simulink model "Uni_Canberra_Inverted_Pendulum"  (R2025b)
settings: Solver=FixedStepDiscrete  StartTime=0  StopTime=50  FixedStep=0.1  RelTol=1e-3
settings Model: Creator=s445788  LastModifiedBy=s445788

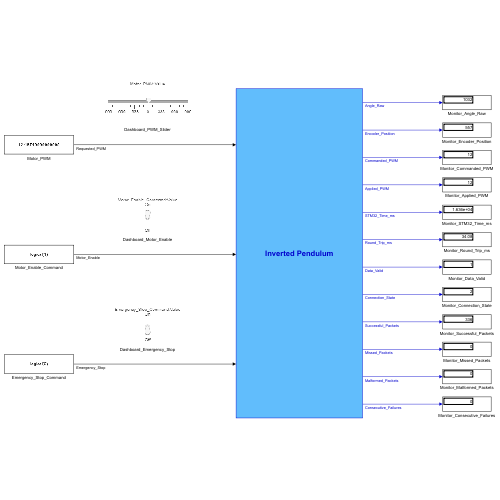
[thumbnail: Simulink's stored preview of the top-level diagram]
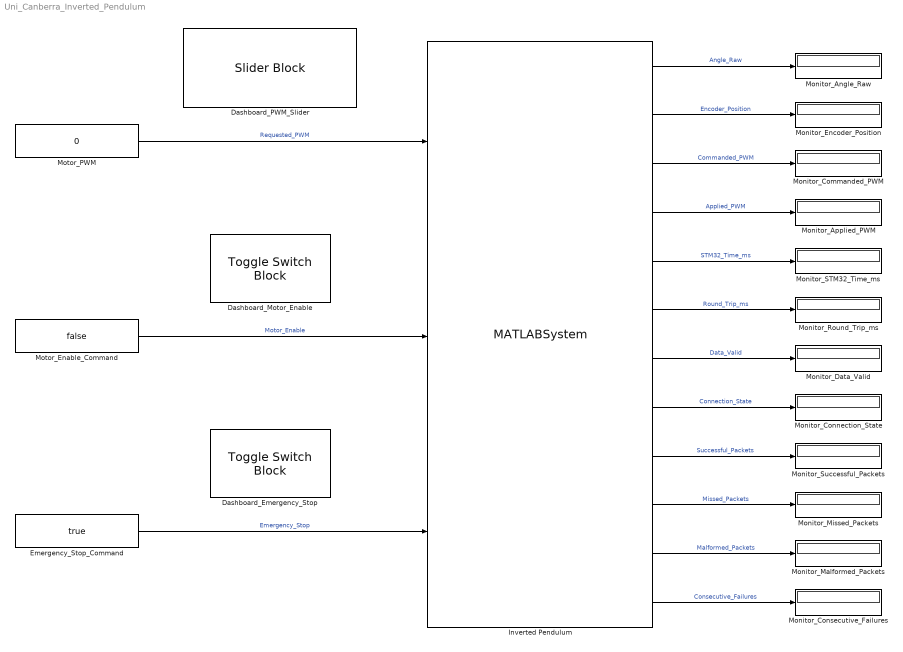
== system Uni_Canberra_Inverted_Pendulum ==
  Dashboard_Emergency_Stop : ToggleSwitchBlock
  Dashboard_Motor_Enable : ToggleSwitchBlock
  Dashboard_PWM_Slider : SliderBlock  ScaleMin=-999  ScaleMax=999
  Emergency_Stop_Command : Constant  Value=true  OutDataTypeStr=boolean  SampleTime=0.1
  Inverted Pendulum : MATLABSystem  System=STM32SerialSystem  Port=COM4  BaudRate=9600  ResponseTimeout=0.75  CommandRetries=1  MotorRefreshPeriod=0.20  SampleTime=0.10  MaximumConsecutiveFailures=3
      mask Type: STM32SerialSystem
  Monitor_Angle_Raw : Display
  Monitor_Applied_PWM : Display
  Monitor_Commanded_PWM : Display
  Monitor_Connection_State : Display
  Monitor_Consecutive_Failures : Display
  Monitor_Data_Valid : Display
  Monitor_Encoder_Position : Display
  Monitor_Malformed_Packets : Display
  Monitor_Missed_Packets : Display
  Monitor_Round_Trip_ms : Display
  Monitor_STM32_Time_ms : Display
  Monitor_Successful_Packets : Display
  Motor_Enable_Command : Constant  Value=false  OutDataTypeStr=boolean  SampleTime=0.1
  Motor_PWM : Constant  Value=0  OutDataTypeStr=double  SampleTime=0.1
  wires:
  Motor_PWM/1 -> Inverted Pendulum/1  "Requested_PWM"
  Motor_Enable_Command/1 -> Inverted Pendulum/2  "Motor_Enable"
  Emergency_Stop_Command/1 -> Inverted Pendulum/3  "Emergency_Stop"
  Inverted Pendulum/1 -> Monitor_Angle_Raw/1  "Angle_Raw"
  Inverted Pendulum/2 -> Monitor_Encoder_Position/1  "Encoder_Position"
  Inverted Pendulum/3 -> Monitor_Commanded_PWM/1  "Commanded_PWM"
  Inverted Pendulum/4 -> Monitor_Applied_PWM/1  "Applied_PWM"
  Inverted Pendulum/5 -> Monitor_STM32_Time_ms/1  "STM32_Time_ms"
  Inverted Pendulum/6 -> Monitor_Round_Trip_ms/1  "Round_Trip_ms"
  Inverted Pendulum/7 -> Monitor_Data_Valid/1  "Data_Valid"
  Inverted Pendulum/8 -> Monitor_Connection_State/1  "Connection_State"
  Inverted Pendulum/9 -> Monitor_Successful_Packets/1  "Successful_Packets"
  Inverted Pendulum/10 -> Monitor_Missed_Packets/1  "Missed_Packets"
  Inverted Pendulum/11 -> Monitor_Malformed_Packets/1  "Malformed_Packets"
  Inverted Pendulum/12 -> Monitor_Consecutive_Failures/1  "Consecutive_Failures"
